simulink model "example_1"  (R2021a)
settings: Solver=VariableStepAuto  StartTime=0.0  StopTime=1  RelTol=1e-3
settings Model: Creator=YasserNet  LastModifiedBy=YasserNet

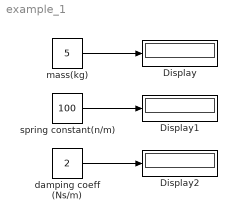
== system example_1 ==
  Display : Display
  Display1 : Display
  Display2 : Display
  damping coeff (Ns/m) : Constant  Value=2
  mass(kg) : Constant  Value=5
  spring constant(n/m) : Constant  Value=100
  wires:
  damping coeff (Ns/m)/1 -> Display2/1
  spring constant(n/m)/1 -> Display1/1
  mass(kg)/1 -> Display/1
